simulink model "MicrogridVessel"  (R2020b)
settings: Solver=FixedStepAuto  StartTime=0.0  StopTime=60*60  FixedStep=Ts  RelTol=1e-3
model workspace: external: MATLAB File LoadParams.m (data not in the file)
undefined symbols (not defined in the file): DCHigh, DCLow
libraries: fl_lib x2, nesl_utility x2
settings Model: DataDictionary=BusSystem.sldd  PauseTimes=36320  OrderedModelArguments=off  Creator=Administrator  LastModifiedBy=cao2851
settings DataIOCC: ExternalInput=inports_dataset{1}  LoadExternalInput=on  SignalLogging=off  DSMLogging=off  SaveTime=off  ReturnWorkspaceOutputsName=ret
settings DebuggingCC: SignalInfNanChecking=error  AlgebraicLoopMsg=error  UnconnectedLineMsg=error  ModelReferenceExtraNoncontSigs=warning
settings ModelReferenceCC: UpdateModelReferenceTargets=IfOutOfDate
settings SimscapeCC: SimscapeLogSimulationStatistics=on  SimscapeLogToSDI=on  SimscapeLogLimitData=off

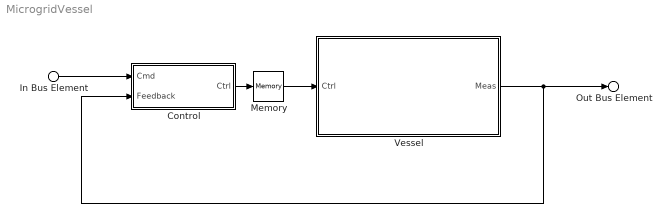
== system MicrogridVessel ==
  In Bus Element : Inport  PortName=Cmd
  Control : Subsystem  TreatAsAtomicUnit=on  SystemSampleTime=1
  Memory : Memory  InheritSampleTime=on
  Vessel : Subsystem
  Out Bus Element : Outport  PortName=Meas
  wires:
  Control/1(Ctrl) -> Memory/1
  Memory/1 -> Vessel/1(Ctrl)
  In Bus Element/1 -> Control/1(Cmd)
  Vessel/1(Meas) -> Out Bus Element/1, Control/2(Feedback)

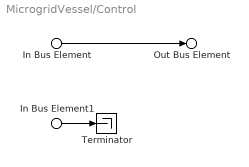
== system MicrogridVessel/Control ==
  In Bus Element : Inport  PortName=Cmd
  In Bus Element1 : Inport  Port=2  PortName=Feedback
  Terminator : Terminator
  Out Bus Element : Outport  PortName=Ctrl
  wires:
  In Bus Element/1 -> Out Bus Element/1
  In Bus Element1/1 -> Terminator/1

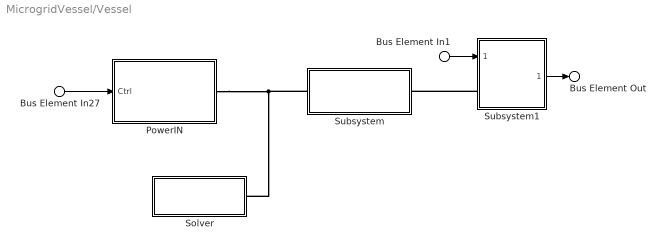
== system MicrogridVessel/Vessel ==
  Bus Element In27 : Inport  PortName=Ctrl  Element=InputVoltage
  Bus Element In1 : Inport  PortName=Ctrl  Element=PowerLoad
  PowerIN : Subsystem
  Solver : Subsystem
  Subsystem : Subsystem  ReferencedSubsystem=Line
  Subsystem1 : Subsystem  ReferencedSubsystem=Load
  Bus Element Out : Outport  PortName=Meas  Element=PowerLoad
  wires:
  Bus Element In27/1 -> PowerIN/1(Ctrl)
  Bus Element In1/1 -> Subsystem1/1
  Subsystem1/1 -> Bus Element Out/1
  connections:
  PowerIN/RConn1 -- Subsystem/LConn1 -- Solver/RConn1
  Subsystem1/LConn1 -- Subsystem/RConn1

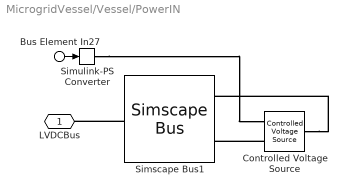
== system MicrogridVessel/Vessel/PowerIN ==
  Bus Element In27 : Inport  PortName=Ctrl  Element=LoadSetpoint
  Controlled Voltage Source : fl_lib/Electrical/Electrical Sources/Controlled Voltage Source
  Simscape Bus1 : SimscapeBus  HierarchyStrings=DCHigh;DCLow
  Simulink-PS Converter : nesl_utility/Simulink-PS Converter  PhysicalDomain=network_engine_domain  SubClassName=ps_input  LeftPortType=input  RightPortType=output  PseudoPeriodic=off  Frequencies=[]  NoiseDistribution=none  NoiseParameters=[]  Unit=1  AffineConversion=off  FilteringAndDerivatives=provide  SimscapeFilterOrder=1  InputFilterTimeConstant=0.001  UdotUserProvided=0
  LVDCBus : PMIOPort  Side=Right
  wires:
  Bus Element In27/1 -> Simulink-PS Converter/1
  connections:
  Simscape Bus1/RConn1 -- LVDCBus/RConn1
  Simulink-PS Converter/RConn1 -- Controlled Voltage Source/RConn1
  Controlled Voltage Source/LConn1 -- Simscape Bus1/LConn1
  Controlled Voltage Source/RConn2 -- Simscape Bus1/LConn2

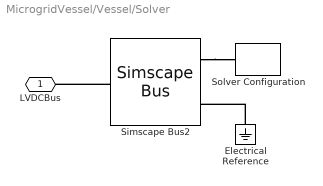
== system MicrogridVessel/Vessel/Solver ==
  Electrical Reference : fl_lib/Electrical/Electrical Elements/Electrical Reference
  Simscape Bus2 : SimscapeBus  HierarchyStrings=DCHigh;DCLow
  Solver Configuration : nesl_utility/Solver Configuration  PhysicalDomain=network_engine_domain  SubClassName=solver  LeftPortType=input  RightPortType=generic  Tones=[]  Harmonics=[]  SimulateNoise=off  Profile=off  UseLocalSampling=off  EnableSwitchedLinearOptims=on  FrequencyDomain=off  UseCCode=off  RelTol=0.001  AbsTol=1e-06  MinStep=1e-09  ToWorkspace=off  RevertToSquareIcSolve=off  NumHomotopyIterations=100  PhasorMode=off  PhasorModeNumHarmonics=1  DoDC=off  ResidualTolerance=1e-09  UseLocalSolver=on  LocalSolverChoice=NE_BACKWARD_EULER_ADVANCER  LocalSolverSampleTime=Ts  DoFixedCost=on  MaxNonlinIter=3  MaxModeIter=2  ComputeImpulses=off  ImpulseIterations=2  LinearAlgebra=auto  EquationFormulation=NE_TIME_EF  DelaysMemoryBudget=1024  AutomaticFiltering=off  FilteringTimeConstant=0.001  PartitionStorageMethod=AS_NEEDED  PartitionMemoryBudget=1024  PartitionMethod=ROBUST
      settings: SourceProductBaseCode=PW,SS
  LVDCBus : PMIOPort  Side=Right
  connections:
  Simscape Bus2/RConn1 -- LVDCBus/RConn1
  Simscape Bus2/LConn1 -- Solver Configuration/RConn1
  Electrical Reference/LConn1 -- Simscape Bus2/LConn2
